simulink model "Controller"  (R2020a)
settings: Solver=FixedStepDiscrete  StartTime=0.0  StopTime=inf  FixedStep=Ts  RelTol=1e-3
values from neighbouring files (symbols this model uses):
  driver_decel = 4.0    (= 4)    [helperLFSetUp.m]
  FB_decel = 9.8    [helperLFSetUp.m]
  Fyf1 = zeros(1,57)    [FyfLookup05.m]
  headwayOffset = 3.7    [helperLFSetUp.m]
  m = 2272    [FyfLookup05.m]    (also in helperLFSetUp.m)
  max_dc = -10    [helperLFSetUp.m]
  PB1_decel = 3.8    [helperLFSetUp.m]
  PB2_decel = 5.3    [helperLFSetUp.m]
  posSelector = [1,0,0,0,0,0; 0,0,1,0,0,0]    [helperLFSetUp.m]
  PredictionHorizon = 30    [helperLFSetUp.m]
  PredictionHorizon1 = 60    [helperLFSetUp.m]
  SlipAngle1 = -SlipAngle1    [FyfLookup05.m]
  time_gap = 1.5    [helperLFSetUp.m]
  timeMargin = 0    [helperLFSetUp.m]
  timeToReact = 1.2    [helperLFSetUp.m]
  Ts = 0.1    [helperLFSetUp.m]
libraries: drivinglib x4, simulink x2, mpcadaslib x1, mpclib x1, simulink_extras x1
(part 2 of 2)

== matlab function Controller/Integrated Controller/Integrated Steering Controller/Successive Linearizer2 ==
  data: A output size=[4,4,PredictionHorizon1+1]; xk input size=[4,1]; moves input; B output size=[4,6,PredictionHorizon1+1]; C output size=[4,4,PredictionHorizon1+1]; D output size=[4,6,PredictionHorizon1+1]; U output size=[6,1,PredictionHorizon1+1]; Y output size=[4,1,PredictionHorizon1+1]; X output size=[4,1,PredictionHorizon1+1]; DX output size=[4,1,PredictionHorizon1+1]; Vx input size=1; ks input; PredictionHorizon1 parameter size=1; DK output; Ts parameter size=1; PredictionHorizon parameter
function [A,B,C,D,U,Y,X,DX,DK] = fcn(xk,moves,Vx,ks,PredictionHorizon1, Ts, PredictionHorizon)
%sucessive updates the LTI plant model required by adaptive MPC controller

% LTV MPC requires p+1 linearizations from k to k+p
Steps = PredictionHorizon1 + 1; % having the number of Steps models
% Initialize outputs
A = zeros(4,4,Steps);
B = zeros(4,6,Steps);
C = zeros(4,4,Steps);
D = zeros(4,6,Steps);
U = zeros(6,1,Steps);
Y = zeros(4,1,Steps);
X = zeros(4,1,Steps);
DX = zeros(4,1,Steps);
DK = zeros(Steps,4); % the constant matrix in the model considered as measured disturbance

% Obtain time varying linear models via successive linearization
for ct = 1:Steps    
    % curveture in next step (but ks only has 31, PredictionHorizon=30+1)
    % assume 32-Steps remain same to the 31th
    if ct > PredictionHorizon+1
        ksk = ks(end);
    else
        ksk = ks(ct);
    end
    % since we don't have u(k) ... u(k+p) at the time of linearization,
    % previous optimal sequence u(k-1) ... u(k+p-1) is used instead.
    if ct>length(moves)
        uk = moves(Steps,:);
    else
        uk = moves(ct,:);
    end
    uk = uk';
    % analytical linearization (continuous time)
    [Ac, Bc, Cc, Dc, dc] = LateralDynamicsCT05(Vx,ksk,xk); % acquiring new characteristic matrix
    % convert A and B matrices from continuous time to discrete time
    % augmenting the model to be in the form of dotX=A*x+B*u while u=[u;dc]
    Aca = Ac;
    Bca = [Bc eye(4)];
    M = expm([[Aca Bca zeros(4,1)]*Ts;zeros(7,11)]);
    Ak = M(1:4,1:4);    %the discrete matrix A for augmented model
    Bk = M(1:4,5:10);   %the discrete matrix B for augmented model
    %store the state space matrix for ct time step
    A(:,:,ct) = Ak;
    B(:,:,ct) = Bk;
    C(:,:,ct) = Cc;
    D(:,:,ct) = [Dc,zeros(4,4)];  % always be zeros(4,6) in fact
    U(:,:,ct) = [uk;dc];          % measured disturbance dc is input as well
    Y(:,:,ct) = xk;               % output is all of the four states
    X(:,:,ct) = xk;               % four states
    DX(:,:,ct) = Ak*xk+Bk*[uk;dc]-xk;%the states increment
    DK(ct,:) = dc';               % disturbance in this step
    % next prediction step
    xk = DX(:,:,ct)+xk;           %update the states
end
